simulink model "ClarkPark_Test"  (R2025b)
settings: Solver=VariableStepAuto  StartTime=0.0  StopTime=10.0  RelTol=1e-3
libraries: MyPMSMLibrary x1
settings Model: Creator=jff_1  LastModifiedBy=jff_1

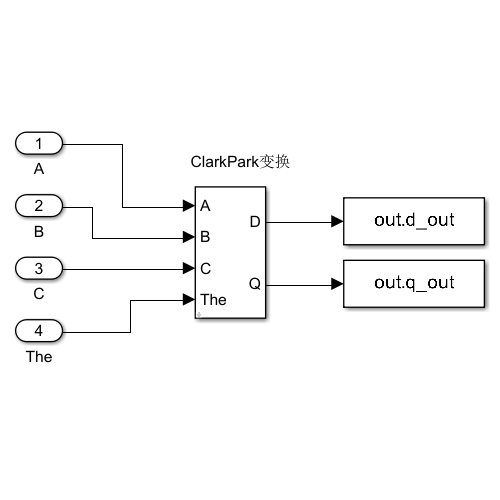
[thumbnail: Simulink's stored preview of the top-level diagram]
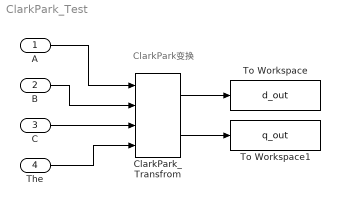
== system ClarkPark_Test ==
  note: ClarkPark变换
  A : Inport
  B : Inport  Port=2
  C : Inport  Port=3
  The : Inport  Port=4
  ClarkPark_Transfrom : MyPMSMLibrary/Transforms/ClarkPark_Transfrom
  To Workspace : ToWorkspace  VariableName=d_out  SampleTime=-1
  To Workspace1 : ToWorkspace  VariableName=q_out  SampleTime=-1
  wires:
  A/1 -> ClarkPark_Transfrom/1
  B/1 -> ClarkPark_Transfrom/2
  C/1 -> ClarkPark_Transfrom/3
  The/1 -> ClarkPark_Transfrom/4
  ClarkPark_Transfrom/1 -> To Workspace/1
  ClarkPark_Transfrom/2 -> To Workspace1/1
